simulink model "Complete_Gesture_Sensor_Model"  (R2022b)
settings: Solver=VariableStepAuto  StartTime=0.0  StopTime=20  RelTol=1e-3
libraries: nesl_utility x9, fl_lib x7, simulink x5, ee_lib x4
settings Model: PacingRate=11  Creator=tonyc  LastModifiedBy=tonyc

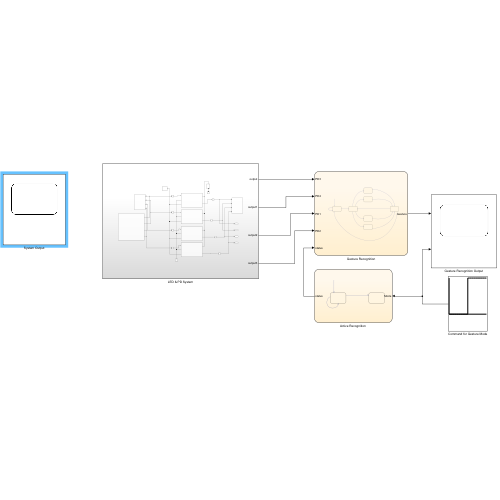
[thumbnail: Simulink's stored preview of the top-level diagram]
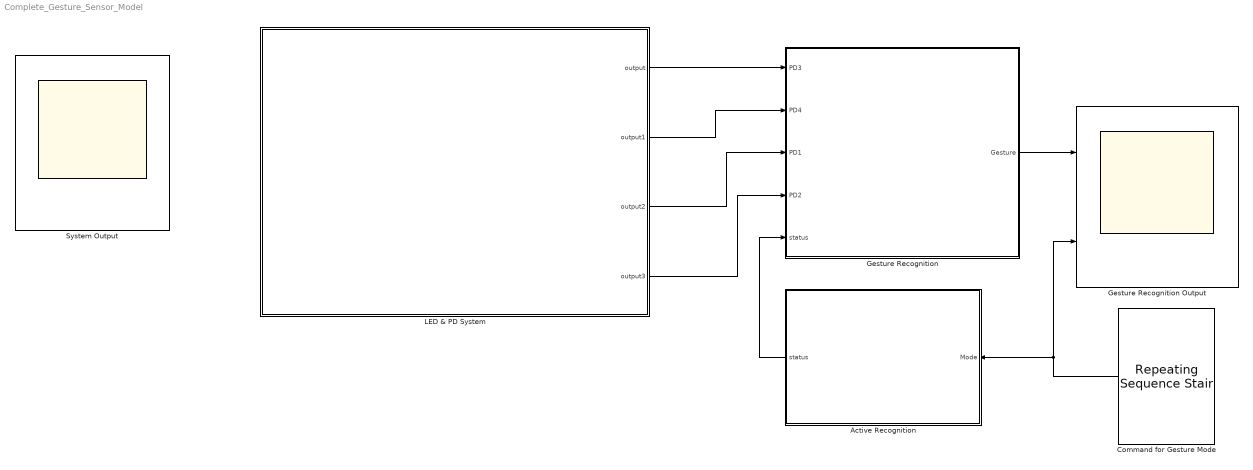
== system Complete_Gesture_Sensor_Model ==
  "Active Recognition " : Stateflow chart  TreatAsAtomicUnit=on
  Command for Gesture Mode : simulink/Sources/Repeating Sequence Stair  OutValues=[ 0 0 0 0 0 0 0 0 0 0 1 1 1 1 1 1 1 1 1 1].'  tsamp=1  OutMin=[]  OutMax=[]  OutDataTypeStr=double  OutputDataTypeScalingMode=double  OutDataType=fixdt(0,8)  ConRadixGroup=Best Precision: Vector-wise  OutScaling=2^-12
  Gesture Recognition : Stateflow chart  TreatAsAtomicUnit=on
  Gesture Recognition Output : Scope  NumInputPorts=2
  LED & PD System : Subsystem
  System Output : Scope
      settings: Floating=on
  wires:
  LED & PD System/1(output) -> Gesture Recognition/1(PD3)
  LED & PD System/2(output1) -> Gesture Recognition/2(PD4)
  LED & PD System/3(output2) -> Gesture Recognition/3(PD1)
  LED & PD System/4(output3) -> Gesture Recognition/4(PD2)
  Command for Gesture Mode/1 -> Gesture Recognition Output/2, "Active Recognition "/1(Mode)
  "Active Recognition "/1(status) -> Gesture Recognition/5(status)
  Gesture Recognition/1(Gesture) -> Gesture Recognition Output/1

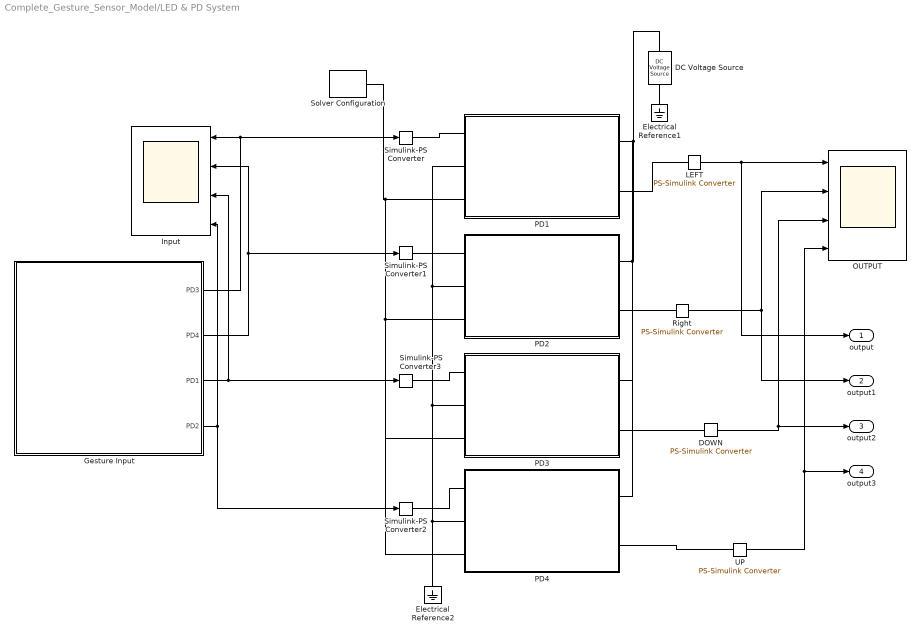
== system Complete_Gesture_Sensor_Model/LED & PD System ==
  DC Voltage Source : fl_lib/Electrical/Electrical Sources/DC Voltage Source  v0=1 V
  DOWN : nesl_utility/PS-Simulink Converter  PhysicalDomain=network_engine_domain  SubClassName=ps_output  LeftPortType=input  RightPortType=output  PseudoPeriodic=off  Frequencies=[]  VectorFormat=inherit  Unit=inherit  AffineConversion=off
  Electrical Reference1 : fl_lib/Electrical/Electrical Elements/Electrical Reference
  Electrical Reference2 : fl_lib/Electrical/Electrical Elements/Electrical Reference
  Gesture Input : Subsystem
  Input : Scope  NumInputPorts=4
  LEFT : nesl_utility/PS-Simulink Converter  PhysicalDomain=network_engine_domain  SubClassName=ps_output  LeftPortType=input  RightPortType=output  PseudoPeriodic=off  Frequencies=[]  VectorFormat=inherit  Unit=inherit  AffineConversion=off
  OUTPUT : Scope  NumInputPorts=4
  PD1 : Subsystem
  PD2 : Subsystem
  PD3 : Subsystem
  PD4 : Subsystem
  Right : nesl_utility/PS-Simulink Converter  PhysicalDomain=network_engine_domain  SubClassName=ps_output  LeftPortType=input  RightPortType=output  PseudoPeriodic=off  Frequencies=[]  VectorFormat=inherit  Unit=inherit  AffineConversion=off
  Simulink-PS Converter{,1..3} (4 alike) : nesl_utility/Simulink-PS Converter  PhysicalDomain=network_engine_domain  SubClassName=ps_input  LeftPortType=input  RightPortType=output  PseudoPeriodic=off  Frequencies=[]  NoiseDistribution=none  NoiseParameters=[]  Unit=1  AffineConversion=off  FilteringAndDerivatives=provide  SimscapeFilterOrder=1  InputFilterTimeConstant=0.001  UdotUserProvided=0
  Solver Configuration : nesl_utility/Solver Configuration  PhysicalDomain=network_engine_domain  SubClassName=solver  LeftPortType=input  RightPortType=generic  Tones=[]  Harmonics=[]  SimulateNoise=off  Profile=off  UseLocalSampling=off  EnableSwitchedLinearOptims=on  FrequencyDomain=off  UseCCode=off  RelTol=0.001  AbsTol=0.001  MinStep=1e-09  ToWorkspace=off  RevertToSquareIcSolve=off  NumHomotopyIterations=100  PhasorMode=off  PhasorModeNumHarmonics=1  ConsistencySolver=NEWTON_XTOL_AFTER_FTOL  IndexReductionMethod=DerivativeReplacement  DoDC=off  ResidualTolerance=1e-09  ConsistencyTolSource=GLOBAL  ConsistencyAbsTol=0.001  ConsistencyRelTol=0.001  ConsistencyTolFactor=0.001  UseLocalSolver=off  LocalSolverChoice=NE_BACKWARD_EULER_ADVANCER  ResolveIndetEquations=on  FunctionEvalNumThread=1  LocalSolverSampleTime=0.001  DoFixedCost=off  MaxNonlinIter=3  MaxModeIter=2  ComputeImpulses=off  ImpulseIterations=2  LinearAlgebra=auto  LinearAlgebraNumThread=0  EquationFormulation=NE_TIME_EF  DelaysMemoryBudget=1024  AutomaticFiltering=on  FilteringTimeConstant=0.001  PartitionStorageMethod=AS_NEEDED  PartitionMemoryBudget=1024  PartitionMethod=ROBUST
  UP : nesl_utility/PS-Simulink Converter  PhysicalDomain=network_engine_domain  SubClassName=ps_output  LeftPortType=input  RightPortType=output  PseudoPeriodic=off  Frequencies=[]  VectorFormat=inherit  Unit=inherit  AffineConversion=off
  output : Outport
  output1 : Outport  Port=2
  output2 : Outport  Port=3
  output3 : Outport  Port=4
  wires:
  UP/1 -> output3/1, OUTPUT/4
  Gesture Input/1(PD3) -> Simulink-PS Converter/1, Input/1
  LEFT/1 -> output/1, OUTPUT/1
  Gesture Input/2(PD4) -> Simulink-PS Converter1/1, Input/2
  DOWN/1 -> output2/1, OUTPUT/3
  Gesture Input/3(PD1) -> Input/3, Simulink-PS Converter3/1
  Right/1 -> output1/1, OUTPUT/2
  Gesture Input/4(PD2) -> Simulink-PS Converter2/1, Input/4
  connections:
  DC Voltage Source/LConn1 -- PD4/RConn1 -- PD3/RConn1 -- PD2/RConn1 -- PD1/RConn1
  Simulink-PS Converter/RConn1 -- PD1/LConn1
  Electrical Reference1/LConn1 -- DC Voltage Source/RConn1
  PD1/RConn2 -- LEFT/LConn1
  Simulink-PS Converter2/RConn1 -- PD4/LConn1
  Simulink-PS Converter3/RConn1 -- PD3/LConn1
  Simulink-PS Converter1/RConn1 -- PD2/LConn1
  UP/LConn1 -- PD4/RConn2
  DOWN/LConn1 -- PD3/RConn2
  PD2/RConn2 -- Right/LConn1
  PD1/LConn2 -- Electrical Reference2/LConn1 -- PD4/LConn2 -- PD3/LConn2 -- PD2/LConn2
  Solver Configuration/RConn1 -- PD4/LConn3 -- PD3/LConn3 -- PD2/LConn3 -- PD1/LConn3

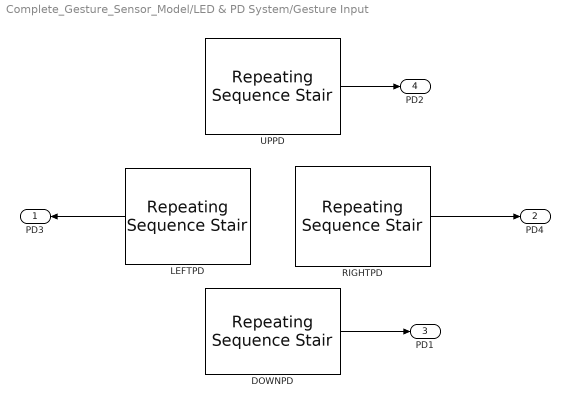
== system Complete_Gesture_Sensor_Model/LED & PD System/Gesture Input ==
  DOWNPD : simulink/Sources/Repeating Sequence Stair  OutValues=100000*[1 1 1 1 1 5 5 5 1 1 1 1 1 5 5 5 1 1 1 1].'  tsamp=1  OutMin=[]  OutMax=[]  OutDataTypeStr=double  OutputDataTypeScalingMode=double  OutDataType=fixdt(0,8)  ConRadixGroup=Best Precision: Vector-wise  OutScaling=2^-12
  LEFTPD : simulink/Sources/Repeating Sequence Stair  OutValues=100000*[1 1 1 1 5 5 5 1 1 1 1 1 1 1 5 5 5 1 1 1].'  tsamp=1  OutMin=[]  OutMax=[]  OutDataTypeStr=double  OutputDataTypeScalingMode=double  OutDataType=fixdt(0,8)  ConRadixGroup=Best Precision: Vector-wise  OutScaling=2^-12
  RIGHTPD : simulink/Sources/Repeating Sequence Stair  OutValues=100000*[1 1 1 1 4.9 4.9 4.9 1 1 1 1 1 1 1 4.9 4.9 4.9 1 1 1].'  tsamp=1  OutMin=[]  OutMax=[]  OutDataTypeStr=double  OutputDataTypeScalingMode=double  OutDataType=fixdt(0,8)  ConRadixGroup=Best Precision: Vector-wise  OutScaling=2^-12
  UPPD : simulink/Sources/Repeating Sequence Stair  OutValues=100000*[1 1 1 5 5 5 1 1 1 1 1 1 1 1 1 5 5 5 1 1].'  tsamp=1  OutMin=[]  OutMax=[]  OutDataTypeStr=double  OutputDataTypeScalingMode=double  OutDataType=fixdt(0,8)  ConRadixGroup=Best Precision: Vector-wise  OutScaling=2^-12
  PD3 : Outport
  PD4 : Outport  Port=2
  PD1 : Outport  Port=3
  PD2 : Outport  Port=4
  wires:
  LEFTPD/1 -> PD3/1
  DOWNPD/1 -> PD1/1
  UPPD/1 -> PD2/1
  RIGHTPD/1 -> PD4/1

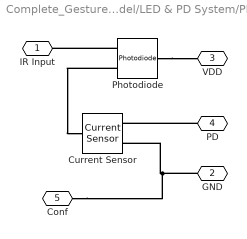
== system Complete_Gesture_Sensor_Model/LED & PD System/PD1 ==
  Current Sensor : fl_lib/Electrical/Electrical Sensors/Current Sensor
  Photodiode : ee_lib/Sensors & Transducers/Photodiode  prmFlux=1  Imeas=25 uA  FluxD=5 W/m^2  G=5e-6 A*m^2/W  prmExp=1  I2=0.1 A  V2=1.3 V  IS=5e-9 A  ec=3  RS=0.1 Ohm  Tmeas=25 degC  C_param=1  CJ=60 pF  CJ0=60 pF  VJ=1 V  Mgrad=0.5  Vvec=[.1, 10, 100] V  Cvec=[45, 3, 6] pF  FC=0.5  T_param=1  IS_T2=2.5e-7 A  I1_T2=0.07 A  V1_T2=1.3 V  Tmeas2=125 degC  EG_param=1  EG=1.11 eV  XTI_param=1  XTI=3  Tdevice=25 degC  i_specify=off  i_priority=None  i=0 A  i_nominal_specify=off  i_nominal_unit=A  i_nominal_value=1  v_specify=off  v_priority=None  v=0 V  v_nominal_specify=off  v_nominal_unit=V  v_nominal_value=1  v_capacitor_specify=off  v_capacitor_priority=High  v_capacitor=0 V  v_capacitor_nominal_specify=off  v_capacitor_nominal_unit=V  v_capacitor_nominal_value=1  thermal_network_parameterization=ee.enum.thermalNetworkTopology.junctionCase  Rth=[0, 10] K/W  Rth_Cauer=[1, 3, 10] K/W  Rth_Foster=[4, 6] K/W  thermal_mass_parameterization=ee.enum.thermalNetwork.timeconstant  thermal_mass=[0, 1] J/K  thermal_mass_Cauer=[1.5, 2, 3] J/K  thermal_mass_Foster=[1.5, 3] J/K  thermal_time_constant=[0, 10] s  thermal_time_constant_Cauer=[1, 3, 10] s  thermal_time_constant_Foster=[6, 18] s  thermal_mass_initial_temperatures=[25, 25] degC  thermal_mass_initial_temperatures_Cauer=[25, 25, 25] degC  steadyState_Foster=simscape.enum.onoff.on  Tvec_initial_Foster=[25, 25, 25, 25] degC
      settings: InternalSimscapePortConfiguration="{\"Bottom\":[],\"Left\":[{\"id\":\"W\",\"label\":\"W\",\"type\":\"input\"},{\"id\":\"p\",\"label\":\"\",\"type\":\"foundation.electrical.electrical\"}],\"Right\":[{\"id\":\"n\",\"label\":\"\",\"type\":\"foundation.electrical.electrical\"}],\"Top\":[]}"
  IR Input : PMIOPort  Side=Left
  GND : PMIOPort  Port=2  Side=Left
  VDD : PMIOPort  Port=3  Side=Right
  PD : PMIOPort  Port=4  Side=Right
  Conf : PMIOPort  Port=5  Side=Left
  connections:
  Photodiode/LConn2 -- Current Sensor/LConn1
  Photodiode/RConn1 -- VDD/RConn1
  Photodiode/LConn1 -- IR Input/RConn1
  PD/RConn1 -- Current Sensor/RConn1
  GND/RConn1 -- Conf/RConn1 -- Current Sensor/RConn2

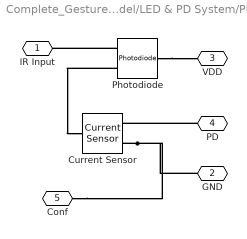
== system Complete_Gesture_Sensor_Model/LED & PD System/PD2 ==
  Current Sensor : fl_lib/Electrical/Electrical Sensors/Current Sensor
  Photodiode : ee_lib/Sensors & Transducers/Photodiode  prmFlux=1  Imeas=25 uA  FluxD=5 W/m^2  G=5e-6 A*m^2/W  prmExp=1  I2=0.1 A  V2=1.3 V  IS=5e-9 A  ec=3  RS=0.1 Ohm  Tmeas=25 degC  C_param=1  CJ=60 pF  CJ0=60 pF  VJ=1 V  Mgrad=0.5  Vvec=[.1, 10, 100] V  Cvec=[45, 3, 6] pF  FC=0.5  T_param=1  IS_T2=2.5e-7 A  I1_T2=0.07 A  V1_T2=1.3 V  Tmeas2=125 degC  EG_param=1  EG=1.11 eV  XTI_param=1  XTI=3  Tdevice=25 degC  i_specify=off  i_priority=None  i=0 A  i_nominal_specify=off  i_nominal_unit=A  i_nominal_value=1  v_specify=off  v_priority=None  v=0 V  v_nominal_specify=off  v_nominal_unit=V  v_nominal_value=1  v_capacitor_specify=off  v_capacitor_priority=High  v_capacitor=0 V  v_capacitor_nominal_specify=off  v_capacitor_nominal_unit=V  v_capacitor_nominal_value=1  thermal_network_parameterization=ee.enum.thermalNetworkTopology.junctionCase  Rth=[0, 10] K/W  Rth_Cauer=[1, 3, 10] K/W  Rth_Foster=[4, 6] K/W  thermal_mass_parameterization=ee.enum.thermalNetwork.timeconstant  thermal_mass=[0, 1] J/K  thermal_mass_Cauer=[1.5, 2, 3] J/K  thermal_mass_Foster=[1.5, 3] J/K  thermal_time_constant=[0, 10] s  thermal_time_constant_Cauer=[1, 3, 10] s  thermal_time_constant_Foster=[6, 18] s  thermal_mass_initial_temperatures=[25, 25] degC  thermal_mass_initial_temperatures_Cauer=[25, 25, 25] degC  steadyState_Foster=simscape.enum.onoff.on  Tvec_initial_Foster=[25, 25, 25, 25] degC
      settings: InternalSimscapePortConfiguration="{\"Bottom\":[],\"Left\":[{\"id\":\"W\",\"label\":\"W\",\"type\":\"input\"},{\"id\":\"p\",\"label\":\"\",\"type\":\"foundation.electrical.electrical\"}],\"Right\":[{\"id\":\"n\",\"label\":\"\",\"type\":\"foundation.electrical.electrical\"}],\"Top\":[]}"
  IR Input : PMIOPort  Side=Left
  GND : PMIOPort  Port=2  Side=Left
  VDD : PMIOPort  Port=3  Side=Right
  PD : PMIOPort  Port=4  Side=Right
  Conf : PMIOPort  Port=5  Side=Left
  connections:
  Photodiode/LConn2 -- Current Sensor/LConn1
  Photodiode/RConn1 -- VDD/RConn1
  Photodiode/LConn1 -- IR Input/RConn1
  PD/RConn1 -- Current Sensor/RConn1
  Current Sensor/RConn2 -- Conf/RConn1 -- GND/RConn1

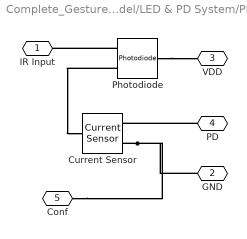
== system Complete_Gesture_Sensor_Model/LED & PD System/PD3 ==
  Current Sensor : fl_lib/Electrical/Electrical Sensors/Current Sensor
  Photodiode : ee_lib/Sensors & Transducers/Photodiode  prmFlux=1  Imeas=25 uA  FluxD=5 W/m^2  G=5e-6 A*m^2/W  prmExp=1  I2=0.1 A  V2=1.3 V  IS=5e-9 A  ec=3  RS=0.1 Ohm  Tmeas=25 degC  C_param=1  CJ=60 pF  CJ0=60 pF  VJ=1 V  Mgrad=0.5  Vvec=[.1, 10, 100] V  Cvec=[45, 3, 6] pF  FC=0.5  T_param=1  IS_T2=2.5e-7 A  I1_T2=0.07 A  V1_T2=1.3 V  Tmeas2=125 degC  EG_param=1  EG=1.11 eV  XTI_param=1  XTI=3  Tdevice=25 degC  i_specify=off  i_priority=None  i=0 A  i_nominal_specify=off  i_nominal_unit=A  i_nominal_value=1  v_specify=off  v_priority=None  v=0 V  v_nominal_specify=off  v_nominal_unit=V  v_nominal_value=1  v_capacitor_specify=off  v_capacitor_priority=High  v_capacitor=0 V  v_capacitor_nominal_specify=off  v_capacitor_nominal_unit=V  v_capacitor_nominal_value=1  thermal_network_parameterization=ee.enum.thermalNetworkTopology.junctionCase  Rth=[0, 10] K/W  Rth_Cauer=[1, 3, 10] K/W  Rth_Foster=[4, 6] K/W  thermal_mass_parameterization=ee.enum.thermalNetwork.timeconstant  thermal_mass=[0, 1] J/K  thermal_mass_Cauer=[1.5, 2, 3] J/K  thermal_mass_Foster=[1.5, 3] J/K  thermal_time_constant=[0, 10] s  thermal_time_constant_Cauer=[1, 3, 10] s  thermal_time_constant_Foster=[6, 18] s  thermal_mass_initial_temperatures=[25, 25] degC  thermal_mass_initial_temperatures_Cauer=[25, 25, 25] degC  steadyState_Foster=simscape.enum.onoff.on  Tvec_initial_Foster=[25, 25, 25, 25] degC
      settings: InternalSimscapePortConfiguration="{\"Bottom\":[],\"Left\":[{\"id\":\"W\",\"label\":\"W\",\"type\":\"input\"},{\"id\":\"p\",\"label\":\"\",\"type\":\"foundation.electrical.electrical\"}],\"Right\":[{\"id\":\"n\",\"label\":\"\",\"type\":\"foundation.electrical.electrical\"}],\"Top\":[]}"
  IR Input : PMIOPort  Side=Left
  GND : PMIOPort  Port=2  Side=Left
  VDD : PMIOPort  Port=3  Side=Right
  PD : PMIOPort  Port=4  Side=Right
  Conf : PMIOPort  Port=5  Side=Left
  connections:
  Photodiode/LConn2 -- Current Sensor/LConn1
  Photodiode/RConn1 -- VDD/RConn1
  Photodiode/LConn1 -- IR Input/RConn1
  PD/RConn1 -- Current Sensor/RConn1
  Current Sensor/RConn2 -- Conf/RConn1 -- GND/RConn1

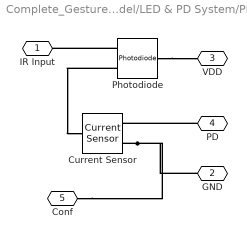
== system Complete_Gesture_Sensor_Model/LED & PD System/PD4 ==
  Current Sensor : fl_lib/Electrical/Electrical Sensors/Current Sensor
  Photodiode : ee_lib/Sensors & Transducers/Photodiode  prmFlux=1  Imeas=25 uA  FluxD=5 W/m^2  G=5e-6 A*m^2/W  prmExp=1  I2=0.1 A  V2=1.3 V  IS=5e-9 A  ec=3  RS=0.1 Ohm  Tmeas=25 degC  C_param=1  CJ=60 pF  CJ0=60 pF  VJ=1 V  Mgrad=0.5  Vvec=[.1, 10, 100] V  Cvec=[45, 3, 6] pF  FC=0.5  T_param=1  IS_T2=2.5e-7 A  I1_T2=0.07 A  V1_T2=1.3 V  Tmeas2=125 degC  EG_param=1  EG=1.11 eV  XTI_param=1  XTI=3  Tdevice=25 degC  i_specify=off  i_priority=None  i=0 A  i_nominal_specify=off  i_nominal_unit=A  i_nominal_value=1  v_specify=off  v_priority=None  v=0 V  v_nominal_specify=off  v_nominal_unit=V  v_nominal_value=1  v_capacitor_specify=off  v_capacitor_priority=High  v_capacitor=0 V  v_capacitor_nominal_specify=off  v_capacitor_nominal_unit=V  v_capacitor_nominal_value=1  thermal_network_parameterization=ee.enum.thermalNetworkTopology.junctionCase  Rth=[0, 10] K/W  Rth_Cauer=[1, 3, 10] K/W  Rth_Foster=[4, 6] K/W  thermal_mass_parameterization=ee.enum.thermalNetwork.timeconstant  thermal_mass=[0, 1] J/K  thermal_mass_Cauer=[1.5, 2, 3] J/K  thermal_mass_Foster=[1.5, 3] J/K  thermal_time_constant=[0, 10] s  thermal_time_constant_Cauer=[1, 3, 10] s  thermal_time_constant_Foster=[6, 18] s  thermal_mass_initial_temperatures=[25, 25] degC  thermal_mass_initial_temperatures_Cauer=[25, 25, 25] degC  steadyState_Foster=simscape.enum.onoff.on  Tvec_initial_Foster=[25, 25, 25, 25] degC
      settings: InternalSimscapePortConfiguration="{\"Bottom\":[],\"Left\":[{\"id\":\"W\",\"label\":\"W\",\"type\":\"input\"},{\"id\":\"p\",\"label\":\"\",\"type\":\"foundation.electrical.electrical\"}],\"Right\":[{\"id\":\"n\",\"label\":\"\",\"type\":\"foundation.electrical.electrical\"}],\"Top\":[]}"
  IR Input : PMIOPort  Side=Left
  GND : PMIOPort  Port=2  Side=Left
  VDD : PMIOPort  Port=3  Side=Right
  PD : PMIOPort  Port=4  Side=Right
  Conf : PMIOPort  Port=5  Side=Left
  connections:
  Photodiode/LConn2 -- Current Sensor/LConn1
  Photodiode/RConn1 -- VDD/RConn1
  Photodiode/LConn1 -- IR Input/RConn1
  PD/RConn1 -- Current Sensor/RConn1
  Current Sensor/RConn2 -- Conf/RConn1 -- GND/RConn1

== stateflow chart Complete_Gesture_Sensor_Model/Active Recognition  ==
  state Idle
  state Start
  (default) -> Idle
  Idle -> Start [order 1] : [Mode==1]{status=1}
  Idle -> Idle [order 2] : [Mode==0]{status=0}
  data: status output; Mode input

== stateflow chart Complete_Gesture_Sensor_Model/Gesture Recognition ==
  state Up
  state Down
  state Sleep
  state Awake
  state Return
  state Right
  state Left
  Up -> Return : [after(5,sec)]{NextR=1;Gesture=0}
  Awake -> Up [order 1] : [PD1>2&&PD2<2&&PD3>2&&PD4>2]{Gesture=1}
  (default) -> Sleep : {Gesture=0;NextR=0;Continue=0}
  Awake -> Down [order 2] : [PD1<2&&PD2>2&&PD3>2&&PD4>2]{Gesture=2}
  Down -> Return : [after(5,sec)]{NextR=1;Gesture=0}
  Sleep -> Sleep [order 2] : [status==0]
  Sleep -> Awake [order 1] : [status == 1]
  Return -> Awake [order 1] : [Continue==0&&NextR==1]{NextR=0}
  Return -> Sleep [order 2] : [Continue==1]{NextR=0}
  Awake -> Left [order 3] : [PD1>2&&PD2>2&&PD3<2&&PD4>2]{Gesture=3}
  Awake -> Right [order 4] : [PD1>2&&PD2>2&&PD3>2&&PD4<2]{Gesture=4}
  Right -> Return : [after(5,sec)]{NextR=1;Gesture=0}
  Left -> Return : [after(5,sec)]{NextR=1;Gesture=0}
  data: PD3 input; PD4 input; PD1 input; PD2 input; Gesture output; status input; NextR local; t local; Continue local double
